simulink model "FSAC2021_V1_Running"  (R2014a)
settings: Solver=FixedStepDiscrete  StartTime=0.0  StopTime=inf  FixedStep=0.0005  RelTol=1e-3
model workspace (MAT data in the model file):
  MCOS : class17 (value not decoded)
  MCOS : class17 (value not decoded)
  MCOS : class17 (value not decoded)
  MCOS : class17 (value not decoded)
  MCOS : class17 (value not decoded)
  MCOS : class17 (value not decoded)
  MCOS : class17 (value not decoded)
  MCOS : class17 (value not decoded)
  MCOS : class17 (value not decoded)
  MCOS : class17 (value not decoded)
  MCOS : class17 (value not decoded)
  MCOS : class17 (value not decoded)
  MCOS : class17 (value not decoded)
  MCOS : class17 (value not decoded)
  MCOS : class17 (value not decoded)
  MCOS : class17 (value not decoded)
  MCOS : class17 (value not decoded)
  MCOS : class17 (value not decoded)
  MCOS : class17 (value not decoded)
  BUZZER_START = 1
  MCOS : class17 (value not decoded)
  MCOS : class17 (value not decoded)
  MCOS : class17 (value not decoded)
  MCOS : class17 (value not decoded)
  MCOS : class17 (value not decoded)
  MCOS : class17 (value not decoded)
  MCOS : class17 (value not decoded)
  MCOS : class17 (value not decoded)
  MCOS : class17 (value not decoded)
  MCOS : class17 (value not decoded)
  MCOS : class17 (value not decoded)
  MCOS : class17 (value not decoded)
  MCOS : class17 (value not decoded)
  MCOS : class17 (value not decoded)
  MCOS : class17 (value not decoded)
  MCOS : class17 (value not decoded)
  MCOS : class17 (value not decoded)
  MCOS : class17 (value not decoded)
  MCOS : class17 (value not decoded)
  MCOS : class17 (value not decoded)
  MCOS : class17 (value not decoded)
  MCOS : class17 (value not decoded)
  MCOS : class17 (value not decoded)
  MCOS : class17 (value not decoded)
  MCOS : class17 (value not decoded)
  MCOS : class17 (value not decoded)
  MCOS : class17 (value not decoded)
  MCOS : class17 (value not decoded)
  MCOS : class17 (value not decoded)
  MCOS : class17 (value not decoded)
  MCOS : class17 (value not decoded)
  MCOS : class17 (value not decoded)
  MCOS : class17 (value not decoded)
  MCOS : class17 (value not decoded)
  MCOS : class17 (value not decoded)
  MCOS : class17 (value not decoded)
  MCOS : class17 (value not decoded)
  MCOS : class17 (value not decoded)
  Brake = 11
  MCOS : class17 (value not decoded)
  MCOS : class17 (value not decoded)
  MCOS : class17 (value not decoded)
  MCOS : class17 (value not decoded)
  MCOS : class17 (value not decoded)
  MCOS : class17 (value not decoded)
  MCOS : class17 (value not decoded)
  MCOS : class17 (value not decoded)
  Sensor_Acc_b = 101.85
  Sensor_Acc_k = -0.0185
  Str_Sen_Orig_Angle = -341
  MCOS : class17 (value not decoded)
  Tire_D = 0.47
  T = 0.05
libraries: simulink x402, ec55xxlib x134
(part 4 of 17)

== system FSAC2021_V1_Running/CAN_SEND/Subsystem1/MOTEC_CONTROL ==
  Fault_Reset_in : Inport
  Position_set_in : Inport  Port=2
  New_Pos_Set_in : Inport  Port=3
  Halt_Ctrl_in : Inport  Port=4
  Abs_or_Rel_Ctrl_in : Inport  Port=5
  Switch_On_Ctrl_in : Inport  Port=6
  Quick_Stop_Ctrl_in : Inport  Port=7
  Enable_Voltage_Ctrl_in : Inport  Port=8
  Enable_Operation_Ctrl_in : Inport  Port=9
  function : TriggerPort  TriggerType=function-call
  Abs_or_Rel_Ctrl : Subsystem
  Conv{1..6} (6 alike) : DataTypeConversion
  Enable_Operation_Ctrl : Subsystem
  Enable_Voltage_Ctrl : Subsystem
  Fault_Reset : Subsystem
  Halt_Ctrl : Subsystem
  MOTEC_CONTROL_mux : Mux  Inputs=6
  New_Pos_Set : Subsystem
  Position_set : Subsystem
  Quick_Stop_Ctrl : Subsystem
  Switch_On_Ctrl : Subsystem
  or1 : simulink/Logic and Bit Operations/Bitwise Operator  logicop=OR  UseBitMask=off  NumInputPorts=7  BitMask=bin2dec('11011001')  BitMaskRealWorld=Stored Integer
  output : Outport
  wires:
  MOTEC_CONTROL_mux/1 -> output/1
  Fault_Reset/1(output1) -> or1/1
  New_Pos_Set/1(output1) -> or1/3
  Abs_or_Rel_Ctrl/1(output1) -> or1/5
  Switch_On_Ctrl/1(output1) -> or1/6
  Quick_Stop_Ctrl/1(output1) -> or1/7
  Enable_Voltage_Ctrl/1(output1) -> or1/2
  Enable_Operation_Ctrl/1(output1) -> or1/4
  or1/1 -> Conv1/1
  Conv1/1 -> MOTEC_CONTROL_mux/1
  Halt_Ctrl/1(output2) -> Conv2/1
  Conv2/1 -> MOTEC_CONTROL_mux/2
  Position_set/1(output3) -> Conv3/1
  Conv3/1 -> MOTEC_CONTROL_mux/3
  Position_set/2(output4) -> Conv4/1
  Conv4/1 -> MOTEC_CONTROL_mux/4
  Position_set/3(output5) -> Conv5/1
  Conv5/1 -> MOTEC_CONTROL_mux/5
  Position_set/4(output6) -> Conv6/1
  Conv6/1 -> MOTEC_CONTROL_mux/6
  Fault_Reset_in/1 -> Fault_Reset/1(Fault_Reset)
  Position_set_in/1 -> Position_set/1(Position_set)
  New_Pos_Set_in/1 -> New_Pos_Set/1(New_Pos_Set)
  Halt_Ctrl_in/1 -> Halt_Ctrl/1(Halt_Ctrl)
  Abs_or_Rel_Ctrl_in/1 -> Abs_or_Rel_Ctrl/1(Abs_or_Rel_Ctrl)
  Switch_On_Ctrl_in/1 -> Switch_On_Ctrl/1(Switch_On_Ctrl)
  Quick_Stop_Ctrl_in/1 -> Quick_Stop_Ctrl/1(Quick_Stop_Ctrl)
  Enable_Voltage_Ctrl_in/1 -> Enable_Voltage_Ctrl/1(Enable_Voltage_Ctrl)
  Enable_Operation_Ctrl_in/1 -> Enable_Operation_Ctrl/1(Enable_Operation_Ctrl)

== system FSAC2021_V1_Running/CAN_SEND/Subsystem1/MOTEC_ENCODER1 ==
  Str_Encoder1_in : Inport
  Str_Encoder2_in : Inport  Port=2
  Str_Encoder3_in : Inport  Port=3
  Str_Encoder4_in : Inport  Port=4
  Str_Encoder5_in : Inport  Port=5
  Str_Encoder6_in : Inport  Port=6
  function : TriggerPort  TriggerType=function-call
  Conv{1..6} (6 alike) : DataTypeConversion
  MOTEC_ENCODER_mux : Mux  Inputs=6
  Str_Encoder1 : Subsystem
  Str_Encoder2 : Subsystem
  Str_Encoder3 : Subsystem
  Str_Encoder4 : Subsystem
  Str_Encoder5 : Subsystem
  Str_Encoder6 : Subsystem
  output : Outport
  wires:
  MOTEC_ENCODER_mux/1 -> output/1
  Str_Encoder1/1(output1) -> Conv1/1
  Conv1/1 -> MOTEC_ENCODER_mux/1
  Str_Encoder2/1(output2) -> Conv2/1
  Conv2/1 -> MOTEC_ENCODER_mux/2
  Conv3/1 -> MOTEC_ENCODER_mux/3
  Str_Encoder4/1(output4) -> Conv4/1
  Conv4/1 -> MOTEC_ENCODER_mux/4
  Str_Encoder5/1(output5) -> Conv5/1
  Conv5/1 -> MOTEC_ENCODER_mux/5
  Str_Encoder6/1(output6) -> Conv6/1
  Conv6/1 -> MOTEC_ENCODER_mux/6
  Str_Encoder4_in/1 -> Str_Encoder4/1(Str_Encoder4)
  Str_Encoder6_in/1 -> Str_Encoder6/1(Str_Encoder6)
  Str_Encoder5_in/1 -> Str_Encoder5/1(Str_Encoder5)
  Str_Encoder3_in/1 -> Str_Encoder3/1(Str_Encoder3)
  Str_Encoder2_in/1 -> Str_Encoder2/1(Str_Encoder2)
  Str_Encoder1_in/1 -> Str_Encoder1/1(Str_Encoder1)
  Str_Encoder3/1(output3) -> Conv3/1

== system FSAC2021_V1_Running/CAN_SEND/Subsystem1/MOTEC_NMT ==
  NMT_nodeorder_in : Inport
  NMT_nodectrl_in : Inport  Port=2
  function : TriggerPort  TriggerType=function-call
  Conv1 : DataTypeConversion
  Conv2 : DataTypeConversion
  MOTEC_NMT_mux : Mux  Inputs=2
  NMT_nodectrl : Subsystem
  NMT_nodeorder : Subsystem
  output : Outport
  wires:
  MOTEC_NMT_mux/1 -> output/1
  NMT_nodeorder/1(output1) -> Conv1/1
  Conv1/1 -> MOTEC_NMT_mux/1
  NMT_nodectrl/1(output2) -> Conv2/1
  Conv2/1 -> MOTEC_NMT_mux/2
  NMT_nodeorder_in/1 -> NMT_nodeorder/1(NMT_nodeorder)
  NMT_nodectrl_in/1 -> NMT_nodectrl/1(NMT_nodectrl)

== system FSAC2021_V1_Running/Controller/200ms_Duty/Light_Subsystem ==
  Light_Status : Inport
  "BLINK " : Subsystem  TreatAsAtomicUnit=on
  Data Type Conversion : DataTypeConversion  OutDataTypeStr=uint8
  If : If  IfExpression=u1 == 0  ElseIfExpressions=u1 == 1
  Merge : Merge  Inputs=3
  OFF : Subsystem  TreatAsAtomicUnit=on
  ON : Subsystem  TreatAsAtomicUnit=on
  Light_Output : Outport
  wires:
  ON/1(Out1) -> Merge/1
  Data Type Conversion/1 -> Light_Output/1
  OFF/1(Out1) -> Merge/2
  Merge/1 -> Data Type Conversion/1
  "BLINK "/1(Out1) -> Merge/3
  Light_Status/1 -> If/1
  If/3 -> "BLINK "/Action
  If/1 -> ON/Action
  If/2 -> OFF/Action

== system FSAC2021_V1_Running/Controller/200ms_Duty/Light_Subsystem1 ==
  Light_Status : Inport
  BLINK : Subsystem  TreatAsAtomicUnit=on
  Data Type Conversion : DataTypeConversion  OutDataTypeStr=uint8
  If : If  IfExpression=u1 == 0  ElseIfExpressions=u1 == 1
  Merge : Merge  Inputs=3
  OFF : Subsystem  TreatAsAtomicUnit=on
  ON : Subsystem  TreatAsAtomicUnit=on
  Light_Output : Outport
  wires:
  If/2 -> OFF/Action
  If/1 -> ON/Action
  If/3 -> BLINK/Action
  Light_Status/1 -> If/1
  BLINK/1(Out1) -> Merge/3
  Merge/1 -> Data Type Conversion/1
  OFF/1(Out1) -> Merge/2
  Data Type Conversion/1 -> Light_Output/1
  ON/1(Out1) -> Merge/1

== system FSAC2021_V1_Running/Controller/200ms_Duty/Light_Subsystem2 ==
  Buzzer_Flag : Inport
  Data Type Conversion : DataTypeConversion  OutDataTypeStr=uint8
  EBS_Horn : Subsystem  TreatAsAtomicUnit=on
  If : If  IfExpression=u1 == 0  ElseIfExpressions=u1 == 1
  Merge : Merge  Inputs=3
  Start_Horn : Subsystem  TreatAsAtomicUnit=on
  off : Subsystem  TreatAsAtomicUnit=on
  Buzzer_Pin : Outport
  Buzzer_Overflag : Outport  Port=2
  wires:
  off/1(Out1) -> Merge/1
  Data Type Conversion/1 -> Buzzer_Pin/1
  Start_Horn/1(Out1) -> Merge/2
  Merge/1 -> Data Type Conversion/1
  EBS_Horn/1(Buzzer_Pin) -> Merge/3
  Buzzer_Flag/1 -> If/1
  If/3 -> EBS_Horn/Action
  If/1 -> off/Action
  If/2 -> Start_Horn/Action
  EBS_Horn/2(Buzzer_Overflag) -> Buzzer_Overflag/1

== system FSAC2021_V1_Running/Controller/50ms_Duty/48Battry_Judge ==
  note: 1.OPEN
      | 0.CLOSE
  Str_Sys_Error : Inport
  Brk_Sys_Error : Inport  Port=2
  AS_48V_Relay : Inport  Port=3
  Logical Operator : Logic  AllPortsSameDT=off  OutDataTypeStr=boolean
  Logical Operator2 : Logic  Operator=OR  AllPortsSameDT=off  OutDataTypeStr=boolean
  Logical Operator3 : Logic  Operator=NOT  Inputs=1  AllPortsSameDT=off  OutDataTypeStr=boolean
  Relay_48V_Pin : Outport
  wires:
  AS_48V_Relay/1 -> Logical Operator/2
  Logical Operator/1 -> Relay_48V_Pin/1
  Str_Sys_Error/1 -> Logical Operator2/1
  Brk_Sys_Error/1 -> Logical Operator2/2
  Logical Operator2/1 -> Logical Operator3/1
  Logical Operator3/1 -> Logical Operator/1

== system FSAC2021_V1_Running/Controller/50ms_Duty/EBS_Judge ==
  note: 0 :disable
  note: 1 :armed
  note: 2 :enable
      |
      | 3: No mean
  EBS_GAS_Prs_1_Val : Inport
  EBS_GAS_Prs_2_Val : Inport  Port=2
  Brk_Liquid_Prs_Val : Inport  Port=3
  Constant : Constant  Value=0.4  OutDataTypeStr=single
  Constant1 : Constant  Value=0.4  OutDataTypeStr=single
  Constant2 : Constant  Value=2.8  OutDataTypeStr=single
  Relational Operator : RelationalOperator  Operator=<=  OutDataTypeStr=boolean
  Relational Operator1 : RelationalOperator  Operator=<=  OutDataTypeStr=boolean
  Relational Operator2 : RelationalOperator  Operator=<=  OutDataTypeStr=boolean
  Truth Table : Truth Table  TreatAsAtomicUnit=on
  EBS_Status : Outport
  wires:
  EBS_GAS_Prs_1_Val/1 -> Relational Operator/1
  Constant/1 -> Relational Operator/2
  Constant1/1 -> Relational Operator1/2
  EBS_GAS_Prs_2_Val/1 -> Relational Operator1/1
  Relational Operator/1 -> Truth Table/1(Gas_1_Flag)  "0:No gas;1 Has gas"
  Relational Operator1/1 -> Truth Table/2(Gas_2_Flag)  "0:No gas;1 Has gas"
  Brk_Liquid_Prs_Val/1 -> Relational Operator2/1
  Constant2/1 -> Relational Operator2/2
  Relational Operator2/1 -> Truth Table/3(Liquid_Flag)  "0:No Brk;1 Has Brk"
  Truth Table/1(EBS_Status) -> EBS_Status/1

== system FSAC2021_V1_Running/Controller/50ms_Duty/HV_Judge  ==
  HV_LIGHT : Inport
  HVMS : Inport  Port=2
  ON_OUT : Inport  Port=3
  ON_IN : Inport  Port=4
  Compare_Volt_mv : Inport  Port=5
  Compare To Constant : simulink/Logic and Bit Operations/Compare To Constant  relop=>=  const=2  OutDataTypeStr=boolean
  Data Type Conversion : DataTypeConversion  OutDataTypeStr=uint8
  Logical Operator : Logic  Inputs=3  AllPortsSameDT=off  OutDataTypeStr=boolean
  Logical Operator1 : Logic  Operator=OR  AllPortsSameDT=off  OutDataTypeStr=boolean
  Logical Operator4 : Logic  AllPortsSameDT=off  OutDataTypeStr=boolean
  MeaModule : ec55xxlib/RapidECU_U2/11Calibration/MeaModule  signal=Compare_Voltage
  TS_Flag : Outport
  wires:
  HVMS/1 -> Logical Operator/2
  ON_OUT/1 -> Logical Operator1/1
  Logical Operator1/1 -> Logical Operator/3
  Logical Operator/1 -> Logical Operator4/2
  Logical Operator4/1 -> Data Type Conversion/1
  Data Type Conversion/1 -> TS_Flag/1
  ON_IN/1 -> Logical Operator1/2
  HV_LIGHT/1 -> Logical Operator/1
  Compare To Constant/1 -> MeaModule/1
  MeaModule/1 -> Logical Operator4/1
  Compare_Volt_mv/1 -> Compare To Constant/1

== system FSAC2021_V1_Running/Controller/50ms_Duty/Lights_Select ==
  Visual_Lights_Vetor : Inport
  Visual_Flag : Inport  Port=2
  IMD_Error : Inport  Port=3
  EBS_Error : Inport  Port=4
  BMS_Error : Inport  Port=5
  Demux : Demux  Outputs=3
  Mux : Mux  Inputs=3
  Switch : Switch  Criteria=u2 > Threshold
  IMD_Light_Sts : Outport
  EBS_Light_Sts : Outport  Port=2
  BMS_Light_Sts : Outport  Port=3
  wires:
  BMS_Error/1 -> Mux/3
  Visual_Flag/1 -> Switch/2
  Visual_Lights_Vetor/1 -> Switch/1
  EBS_Error/1 -> Mux/2
  Mux/1 -> Switch/3
  IMD_Error/1 -> Mux/1
  Switch/1 -> Demux/1
  Demux/1 -> IMD_Light_Sts/1
  Demux/2 -> EBS_Light_Sts/1
  Demux/3 -> BMS_Light_Sts/1

== system FSAC2021_V1_Running/Controller/50ms_Duty/R2D_Judge ==
  AS_R2D : Inport
  Acc_Sensor_Error : Inport  Port=2
  Logical Operator : Logic  AllPortsSameDT=off  OutDataTypeStr=boolean
  Logical Operator1 : Logic  Operator=NOT  Inputs=1  AllPortsSameDT=off  OutDataTypeStr=boolean
  R2D_Pin : Outport
  wires:
  Logical Operator/1 -> R2D_Pin/1
  AS_R2D/1 -> Logical Operator/1
  Acc_Sensor_Error/1 -> Logical Operator1/1
  Logical Operator1/1 -> Logical Operator/2

== system FSAC2021_V1_Running/Controller/50ms_Duty/Safety_Relay_Judge ==
  note: 0:Disable
      | 1:Armed
      | 2:Enable
  Finish_State_Safety_Relay : Inport
  Str_Sys_Error : Inport  Port=2
  Brk_Sys_Error : Inport  Port=3
  Sensor_Error : Inport  Port=4
  Node_Lost : Inport  Port=5
  EBS_Failure : Inport  Port=6
  Logical Operator : Logic  Operator=OR  Inputs=6  AllPortsSameDT=off  OutDataTypeStr=boolean
  Safety_Cir_Relay_Pin : Outport
  wires:
  Logical Operator/1 -> Safety_Cir_Relay_Pin/1
  Finish_State_Safety_Relay/1 -> Logical Operator/1
  EBS_Failure/1 -> Logical Operator/6
  Node_Lost/1 -> Logical Operator/5
  Sensor_Error/1 -> Logical Operator/4
  Brk_Sys_Error/1 -> Logical Operator/3
  Str_Sys_Error/1 -> Logical Operator/2

== system FSAC2021_V1_Running/Controller/50ms_Duty/Subsystem ==
  note: TASK:
      | 1、SKIDPAD
      | 2、ACCELERATION
      | 3、TRACKDRIVE
      | 4、BRAKTEST
      | 5、INSPECTION
      | 6、MANUAL_MODE
  Manual_Acc_Cmd : Inport
  AMI_Duty : Inport  Port=2
  IPC_Acc_Cmd : Inport  Port=3
  EBS_Failure : Inport  Port=4
  IPC_Brk_Cmd : Inport  Port=5
  IPC_Str_Cmd : Inport  Port=6
  origin_flag : Inport  Port=7
  ASSI_State : Inport  Port=8
  Allow_Ctr_Flag : Inport  Port=9
  Chart : Stateflow chart  TreatAsAtomicUnit=on
  Compare To Constant : simulink/Logic and Bit Operations/Compare To Constant  relop===  const=1  OutDataTypeStr=boolean
  Compare To Constant1 : simulink/Logic and Bit Operations/Compare To Constant  relop===  const=2  OutDataTypeStr=boolean
  Compare To Constant2 : simulink/Logic and Bit Operations/Compare To Constant  relop===  const=3  OutDataTypeStr=boolean
  Compare To Constant3 : simulink/Logic and Bit Operations/Compare To Constant  relop===  const=1  OutDataTypeStr=boolean
  Compare To Constant4 : simulink/Logic and Bit Operations/Compare To Constant  relop===  const=1  OutDataTypeStr=boolean
  Compare To Constant5 : simulink/Logic and Bit Operations/Compare To Constant  relop=>=  const=3  OutDataTypeStr=boolean
  Constant : Constant
  Data Type Conversion10 : DataTypeConversion  OutDataTypeStr=single
  Data Type Conversion9 : DataTypeConversion  OutDataTypeStr=uint8
  Logical Operator : Logic  Inputs=4  AllPortsSameDT=off  OutDataTypeStr=boolean
  Logical Operator1 : Logic  AllPortsSameDT=off  OutDataTypeStr=boolean
  MeaModule : ec55xxlib/RapidECU_U2/11Calibration/MeaModule  signal=MODE
  MeaModule1 : ec55xxlib/RapidECU_U2/11Calibration/MeaModule  signal=enable
  MeaModule3 : ec55xxlib/RapidECU_U2/11Calibration/MeaModule  signal=ipc_strr
  Merge : Merge  Inputs=3
  Merge1 : Merge
  Subsystem : Subsystem
  Subsystem1 : Subsystem
  Subsystem2 : Subsystem
  Str_Ctr : Outport
  Brk_Ctr : Outport  Port=2
  Mission_Flag : Outport  Port=3
  Acc_Ctr : Outport  Port=4
  wires:
  Data Type Conversion9/1 -> Brk_Ctr/1
  AMI_Duty/1 -> Chart/1(AMI_Duty)
  Chart/1(MODE) -> MeaModule/1
  MeaModule/1 -> Compare To Constant/1, Compare To Constant1/1, Compare To Constant2/1
  Manual_Acc_Cmd/1 -> Subsystem/1(acc)
  Compare To Constant/1 -> Subsystem/Enable
  EBS_Failure/1 -> Subsystem1/2(EBS_Failure)
  IPC_Brk_Cmd/1 -> Subsystem1/3(IPC_Brk_Cmd)
  IPC_Str_Cmd/1 -> Subsystem1/4(IPC_Str_Cmd)
  IPC_Acc_Cmd/1 -> Subsystem1/1(IPC_Acc_Cmd)
  Subsystem1/1(Brk_Cmd) -> Data Type Conversion9/1
  Compare To Constant2/1 -> Logical Operator/1
  Compare To Constant4/1 -> Logical Operator/2
  origin_flag/1 -> Compare To Constant4/1
  Merge1/1 -> Str_Ctr/1
  Logical Operator/1 -> MeaModule1/1
  Subsystem2/1(ACC) -> [Task_Acc]
  Compare To Constant1/1 -> Logical Operator1/1
  Logical Operator1/1 -> Subsystem1/Enable
  Compare To Constant3/1 -> Logical Operator/3
  Constant/1 -> Compare To Constant3/1, Logical Operator1/2
  Subsystem1/3(Acc_Cmd) -> [IPC_Acc_Cmd]
  Subsystem/1(Acc_Cmd) -> [Manual_Acc]
  Data Type Conversion10/1 -> Acc_Ctr/1
  Merge/1 -> Data Type Conversion10/1
  [IPC_Acc_Cmd] -> Merge/1
  [Manual_Acc] -> Merge/2
  [Task_Acc] -> Merge/3
  Subsystem1/2(Str_Cmd) -> [IPC_Str_Cmd]
  Subsystem2/2(SteerCmd) -> [Task_Steer_Cmd]
  [IPC_Str_Cmd] -> MeaModule3/1
  MeaModule1/1 -> Subsystem2/Enable
  MeaModule3/1 -> Merge1/1
  [Task_Steer_Cmd] -> Merge1/2
  Subsystem2/3(Mission_Flag) -> Mission_Flag/1
  Compare To Constant5/1 -> Logical Operator/4
  ASSI_State/1 -> Compare To Constant5/1

== system FSAC2021_V1_Running/Controller/50ms_Duty/Visuality Check ==
  function : TriggerPort  TriggerType=function-call
  Chart : Stateflow chart  TreatAsAtomicUnit=on
  Visual_Lights_Vector : Outport
  Visual_Flag : Outport  Port=2
  wires:
  Chart/1(Visual_Lights) -> Visual_Lights_Vector/1
  Chart/2(Visual_Flag) -> Visual_Flag/1

== system FSAC2021_V1_Running/Controller/BCU_Controller/Brk_Move ==
  Brk_Ctrl_State : Inport
  Brk_Cmd : Inport  Port=2
  Constant : Constant  Value=BRK_ENGAGED
  Constant1 : Constant  Value=BRK_TOZERO
  Constant2 : Constant  Value=BRK_MOVE
  Enabled Subsystem : Subsystem  TreatAsAtomicUnit=on
  Enabled Subsystem1 : Subsystem  TreatAsAtomicUnit=on
  Enabled Subsystem2 : Subsystem  TreatAsAtomicUnit=on
  Equal : RelationalOperator  Operator===  OutDataTypeStr=boolean
  Equal1 : RelationalOperator  Operator===  OutDataTypeStr=boolean
  Equal2 : RelationalOperator  Operator===  OutDataTypeStr=boolean
  Multiport Switch : MultiPortSwitch  DiagnosticForDefault=None
  Brk_Mtr_GoalPos : Outport
  tag scope: Engaged_Angle=global
  wires:
  [Engaged_Angle] -> Enabled Subsystem1/1(Engaged_Angle)
  Enabled Subsystem/2(Engaged_Angle) -> [Engaged_Angle]
  Brk_Cmd/1 -> Enabled Subsystem2/1(Brk_Prop)
  Enabled Subsystem2/1(Move_Pulses) -> Multiport Switch/4
  Enabled Subsystem1/1(ToZero_Pulses) -> Multiport Switch/3
  Enabled Subsystem/1(Engaged_Pulses) -> Multiport Switch/2
  Equal2/1 -> Enabled Subsystem2/Enable
  Equal1/1 -> Enabled Subsystem1/Enable
  Equal/1 -> Enabled Subsystem/Enable
  Constant2/1 -> Equal2/2
  Constant1/1 -> Equal1/2
  Constant/1 -> Equal/2
  Brk_Ctrl_State/1 -> Multiport Switch/1, Equal/1, Equal1/1, Equal2/1
  Multiport Switch/1 -> Brk_Mtr_GoalPos/1

== system FSAC2021_V1_Running/Controller/SteerCtr/Subsystem3 ==
  In1 : Inport
  Constant : Constant  Value=Str_Sen_Orig_Angle  OutDataTypeStr=int16
  Real_steer_angle : Sum  Inputs=+-  OutDataTypeStr=single
  Out1 : Outport
  wires:
  Real_steer_angle/1 -> Out1/1
  In1/1 -> Real_steer_angle/1
  Constant/1 -> Real_steer_angle/2

== system FSAC2021_V1_Running/DIAG/DIAG/Analog_Sensor_Diag ==
  Acc_Lft_Disp_mv : Inport
  Acc_Right_Disp_mv : Inport  Port=2
  Brk_Liquid_Prs_mv : Inport  Port=3
  EBS_GAS_Prs_1_mv : Inport  Port=4
  EBS_GAS_Prs_2_mv : Inport  Port=5
  Chart2 : Stateflow chart  TreatAsAtomicUnit=on
      settings: RTWSystemCode=Reusable function
  Chart3 : Stateflow chart  TreatAsAtomicUnit=on
      settings: RTWSystemCode=Reusable function
  Chart4 : Stateflow chart  TreatAsAtomicUnit=on
      settings: RTWSystemCode=Reusable function
  Chart5 : Stateflow chart  TreatAsAtomicUnit=on
      settings: RTWSystemCode=Reusable function
  Chart6 : Stateflow chart  TreatAsAtomicUnit=on
      settings: RTWSystemCode=Reusable function
  Compare To Constant{,1..4} (5 alike) : simulink/Logic and Bit Operations/Compare To Constant  relop=<=  const=Min  OutDataTypeStr=boolean
  Data Type Conversion{1..5} (5 alike) : DataTypeConversion  OutDataTypeStr=uint8
  Logical Operator8 : Logic  Operator=OR  Inputs=5  AllPortsSameDT=off  OutDataTypeStr=boolean
  MeaModule : ec55xxlib/RapidECU_U2/11Calibration/MeaModule  signal=sensor_erroe
  Acc_Lft_Error : Outport
  Acc_Right_Disp_Error : Outport  Port=2
  Brk_Liquid_Prs_Error : Outport  Port=3
  Sensor_Error : Outport  Port=4
  EBS_GAP_pRS_1_Error : Outport  Port=5
  EBS_GAP_pRS_2_Error : Outport  Port=6
  wires:
  EBS_GAS_Prs_1_mv/1 -> Compare To Constant3/1
  Acc_Lft_Disp_mv/1 -> Compare To Constant/1
  Acc_Right_Disp_mv/1 -> Compare To Constant1/1
  EBS_GAS_Prs_2_mv/1 -> Compare To Constant4/1
  Logical Operator8/1 -> MeaModule/1
  Chart2/1(Debounce) -> Acc_Lft_Error/1, Logical Operator8/1
  Chart3/1(Debounce) -> Acc_Right_Disp_Error/1, Logical Operator8/2
  Chart4/1(Debounce) -> Brk_Liquid_Prs_Error/1, Logical Operator8/3
  Chart5/1(Debounce) -> Logical Operator8/4, EBS_GAP_pRS_1_Error/1
  Chart6/1(Debounce) -> Logical Operator8/5, EBS_GAP_pRS_2_Error/1
  Data Type Conversion1/1 -> Chart2/1(Non_Debounce)
  Data Type Conversion2/1 -> Chart3/1(Non_Debounce)
  Data Type Conversion3/1 -> Chart4/1(Non_Debounce)
  Data Type Conversion4/1 -> Chart5/1(Non_Debounce)
  Data Type Conversion5/1 -> Chart6/1(Non_Debounce)
  Brk_Liquid_Prs_mv/1 -> Compare To Constant2/1
  Compare To Constant1/1 -> Data Type Conversion2/1
  Compare To Constant/1 -> Data Type Conversion1/1
  Compare To Constant2/1 -> Data Type Conversion3/1
  Compare To Constant3/1 -> Data Type Conversion4/1
  Compare To Constant4/1 -> Data Type Conversion5/1
  MeaModule/1 -> Sensor_Error/1

== system FSAC2021_V1_Running/DIAG/DIAG/BMS_Diag ==
  ALM_BATT_OC_Out1 : Inport
  ALM_AUX_FAIL_Out1 : Inport  Port=2
  ALM_BATT_UV_Out1 : Inport  Port=3
  ALM_BATT_OV_Out1 : Inport  Port=4
  ALM_BATT_DT_Out1 : Inport  Port=5
  ALM_BATT_DV_Out1 : Inport  Port=6
  ALM_CELL_TBK_Out1 : Inport  Port=7
  ALM_CELL_IBK_Out1 : Inport  Port=8
  ALM_CELL_UT_Out1 : Inport  Port=9
  ALM_CELL_OT_Out1 : Inport  Port=10
  ALM_CELL_UV_Out1 : Inport  Port=11
  ALM_CELL_OV_Out1 : Inport  Port=12
  ALM_BATT_UC_Out1 : Inport  Port=13
  ALM_PRECHRG_FAIL_Out1 : Inport  Port=14
  ALM_LEAK_OC_Out1 : Inport  Port=15
  ALM_HVREL_FAIL_Out1 : Inport  Port=16
  ALM_HALL_BREAK_Out1 : Inport  Port=17
  ALM_BSU_OFFLINE_Out1 : Inport  Port=18
  ALM_BSU_FAULT_Out1 : Inport  Port=19
  ALM_BMU_FAIL_Out1 : Inport  Port=20
  Data Type Conversion{,1..16,19,22..23} (20 alike) : DataTypeConversion  OutDataTypeStr=boolean  SaturateOnIntegerOverflow=on  RndMeth=Zero
  Data Type Conversion17 : DataTypeConversion  OutDataTypeStr=uint8
  Logical Operator : Logic  Operator=OR  Inputs=20  AllPortsSameDT=off  OutDataTypeStr=boolean
  "BMS_Error " : Outport
  wires:
  ALM_BATT_OC_Out1/1 -> Data Type Conversion/1
  ALM_BATT_DT_Out1/1 -> Data Type Conversion1/1
  ALM_AUX_FAIL_Out1/1 -> Data Type Conversion2/1
  ALM_BATT_UV_Out1/1 -> Data Type Conversion3/1
  ALM_BATT_OV_Out1/1 -> Data Type Conversion4/1
  ALM_CELL_TBK_Out1/1 -> Data Type Conversion5/1
  ALM_CELL_UV_Out1/1 -> Data Type Conversion6/1
  ALM_CELL_UT_Out1/1 -> Data Type Conversion7/1
  ALM_CELL_IBK_Out1/1 -> Data Type Conversion8/1
  ALM_BATT_DV_Out1/1 -> Data Type Conversion9/1
  ALM_CELL_OT_Out1/1 -> Data Type Conversion10/1
  ALM_BATT_UC_Out1/1 -> Data Type Conversion11/1
  ALM_CELL_OV_Out1/1 -> Data Type Conversion12/1
  ALM_PRECHRG_FAIL_Out1/1 -> Data Type Conversion13/1
  ALM_LEAK_OC_Out1/1 -> Data Type Conversion14/1
  ALM_HVREL_FAIL_Out1/1 -> Data Type Conversion15/1
  ALM_HALL_BREAK_Out1/1 -> Data Type Conversion16/1
  ALM_BSU_OFFLINE_Out1/1 -> Data Type Conversion19/1
  ALM_BMU_FAIL_Out1/1 -> Data Type Conversion22/1
  ALM_BSU_FAULT_Out1/1 -> Data Type Conversion23/1
  Data Type Conversion3/1 -> Logical Operator/11
  Data Type Conversion4/1 -> Logical Operator/12
  Data Type Conversion2/1 -> Logical Operator/10
  Data Type Conversion1/1 -> Logical Operator/13
  Data Type Conversion/1 -> Logical Operator/9
  Data Type Conversion11/1 -> Logical Operator/8
  Data Type Conversion9/1 -> Logical Operator/14
  Data Type Conversion5/1 -> Logical Operator/15
  Data Type Conversion22/1 -> Logical Operator/7
  Data Type Conversion23/1 -> Logical Operator/6
  Data Type Conversion8/1 -> Logical Operator/16
  Data Type Conversion16/1 -> Logical Operator/4
  Data Type Conversion7/1 -> Logical Operator/17
  Data Type Conversion19/1 -> Logical Operator/5
  Data Type Conversion10/1 -> Logical Operator/18
  Data Type Conversion15/1 -> Logical Operator/3
  Data Type Conversion6/1 -> Logical Operator/19
  Data Type Conversion14/1 -> Logical Operator/2
  Data Type Conversion13/1 -> Logical Operator/1
  Data Type Conversion12/1 -> Logical Operator/20
  Logical Operator/1 -> Data Type Conversion17/1
  Data Type Conversion17/1 -> "BMS_Error "/1

== system FSAC2021_V1_Running/DIAG/DIAG/Brake_System_Diag ==
  Brake_reg_rw_fault_flag_Out : Inport
  Brake_overheat_prtct_sts_Out : Inport  Port=2
  Brake_overcurrt_prtct_sts_Out : Inport  Port=3
  Brake_lowvolt_prtct_sts_Out : Inport  Port=4
  Brake_hd_fault_sts_Out : Inport  Port=5
  Brake_encoder_fault_sts_Out : Inport  Port=6
  Brake_cmd_fault_flag_Out : Inport  Port=7
  Logical Operator : Logic  Operator=OR  Inputs=7  AllPortsSameDT=off  OutDataTypeStr=boolean
  Brk_Sys_Error : Outport
  wires:
  Brake_cmd_fault_flag_Out/1 -> Logical Operator/7
  Brake_hd_fault_sts_Out/1 -> Logical Operator/5
  Brake_encoder_fault_sts_Out/1 -> Logical Operator/6
  Brake_overheat_prtct_sts_Out/1 -> Logical Operator/2
  Brake_reg_rw_fault_flag_Out/1 -> Logical Operator/1
  Brake_lowvolt_prtct_sts_Out/1 -> Logical Operator/4
  Brake_overcurrt_prtct_sts_Out/1 -> Logical Operator/3
  Logical Operator/1 -> Brk_Sys_Error/1

== system FSAC2021_V1_Running/DIAG/DIAG/CAN_NODE_LOSTCOM ==
  Brake_Node : Inport
  StrSr_Node : Inport  Port=2
  48V_Relay : Inport  Port=3
  RES_Node : Inport  Port=4
  BMS_Node : Inport  Port=5
  Motor_Node : Inport  Port=6
  Motec_Node : Inport  Port=7
  AMI_Node : Inport  Port=8
  ASSI_State : Inport  Port=9
  B_M_S_Check : Subsystem
  Compare To Constant : simulink/Logic and Bit Operations/Compare To Constant  relop=>=  const=3.0  OutDataTypeStr=boolean
  Compare To Constant1 : simulink/Logic and Bit Operations/Compare To Constant  relop=<=  const=5  OutDataTypeStr=boolean
  Constant : Constant
  Constant1 : Constant
  Constant2 : Constant
  Logical Operator : Logic  Inputs=3  AllPortsSameDT=off  OutDataTypeStr=boolean
  Logical Operator1 : Logic  AllPortsSameDT=off  OutDataTypeStr=boolean
  Logical Operator3 : Logic  Operator=NOT  AllPortsSameDT=off  OutDataTypeStr=boolean
  MeaModule : ec55xxlib/RapidECU_U2/11Calibration/MeaModule  signal=Node_Lost
  Subsystem : Subsystem
  Subsystem1 : Subsystem
  Switch : Switch  Criteria=u2 > Threshold
  Switch1 : Switch  Criteria=u2 > Threshold
  Node_Lost_Flag : Outport
  wires:
  Brake_Node/1 -> B_M_S_Check/1(Brake_Node)
  48V_Relay/1 -> Switch/2, B_M_S_Check/Enable
  B_M_S_Check/1(Node_Lost_Flag) -> Switch/1
  Logical Operator3/1 -> MeaModule/1
  Motec_Node/1 -> B_M_S_Check/2(Motec_Node)
  Constant/1 -> B_M_S_Check/3(RES_Node)
  MeaModule/1 -> Node_Lost_Flag/1
  Motor_Node/1 -> Subsystem/1(Motor_Node)
  Subsystem/1(Node_Lost_Flag) -> Switch1/1
  Constant1/1 -> Switch1/3
  Constant2/1 -> Switch/3
  ASSI_State/1 -> Compare To Constant/1, Compare To Constant1/1
  Switch/1 -> Logical Operator/1
  Logical Operator1/1 -> Subsystem/Enable, Switch1/2
  Compare To Constant/1 -> Logical Operator1/1
  Compare To Constant1/1 -> Logical Operator1/2
  Logical Operator/1 -> Logical Operator3/1
  StrSr_Node/1 -> Subsystem1/1(StrSr_Node)
  BMS_Node/1 -> Subsystem1/2(BMS_Node)
  AMI_Node/1 -> Subsystem1/3(AMI_Node)
  Switch1/1 -> Logical Operator/3
  Subsystem1/1(Out1) -> Logical Operator/2

== system FSAC2021_V1_Running/DIAG/DIAG/EBS_Diag ==
  ASSI_State : Inport
  EBS_GAS_Prs_1_Val : Inport  Port=2  OutDataTypeStr=uint16
  EBS_GAS_Prs_2_Val : Inport  Port=3  OutDataTypeStr=uint16
  Truth Table : Truth Table  TreatAsAtomicUnit=on
  EBS_Failuer_Flag : Outport
  wires:
  ASSI_State/1 -> Truth Table/1(ASSI_State)
  Truth Table/1(EBS_Failure_Flag) -> EBS_Failuer_Flag/1
  EBS_GAS_Prs_1_Val/1 -> Truth Table/2(EBS_GAS_Prs_1_Val)
  EBS_GAS_Prs_2_Val/1 -> Truth Table/3(EBS_GAS_Prs_2_Val)

== system FSAC2021_V1_Running/DIAG/DIAG/Res_Diag ==
  RES_SINGNAL : Inport
  ASMS : Inport  Port=2
  MeaModule : ec55xxlib/RapidECU_U2/11Calibration/MeaModule  signal=ASMS_VALUE
  MeaModule1 : ec55xxlib/RapidECU_U2/11Calibration/MeaModule  signal=res_go
  MeaModule2 : ec55xxlib/RapidECU_U2/11Calibration/MeaModule  signal=res_ebs1
  Subsystem : Subsystem
  Res_Go : Outport
  RES_EBS : Outport  Port=2
  wires:
  Subsystem/1(RES_GO) -> MeaModule1/1
  ASMS/1 -> MeaModule/1
  MeaModule/1 -> Subsystem/Enable
  RES_SINGNAL/1 -> Subsystem/1(RES_SINGNAL)
  Subsystem/2(RES_EBS) -> MeaModule2/1
  MeaModule1/1 -> Res_Go/1
  MeaModule2/1 -> RES_EBS/1

== system FSAC2021_V1_Running/DIAG/DIAG/Steer_System_Diag ==
  Str_UnderVolt_Warning_Out : Inport
  Str_System_Error_Out : Inport  Port=2
  Str_Limit_Pos_Alarm_Out : Inport  Port=3
  Str_I2t_Warning_Out : Inport  Port=4
  Str_I2t_Alarm_Out : Inport  Port=5
  Str_Flash_Error_Out : Inport  Port=6
  Str_Encoder_Error_Out : Inport  Port=7
  Str_Curr_Error_Fault_Out : Inport  Port=8
  Str_Spd_Over_Alam_Out : Inport  Port=9
  Str_PwrMod_TempHigh_Warning_Out : Inport  Port=10
  Str_PwrMod_TempHigh_Alarm_Out : Inport  Port=11
  Str_Para_Error_Out : Inport  Port=12
  Str_Overvolt_Warning_Out : Inport  Port=13
  Str_Over_TopCurr_Out : Inport  Port=14
  Str_Over_SpdError_Out : Inport  Port=15
  Str_Over_PosError_Out : Inport  Port=16
  Logical Operator : Logic  Operator=OR  Inputs=16  AllPortsSameDT=off  OutDataTypeStr=boolean
  Str_Sys_Error : Outport
  wires:
  Str_UnderVolt_Warning_Out/1 -> Logical Operator/1
  Str_System_Error_Out/1 -> Logical Operator/2
  Str_Spd_Over_Alam_Out/1 -> Logical Operator/3
  Str_PwrMod_TempHigh_Warning_Out/1 -> Logical Operator/4
  Str_Limit_Pos_Alarm_Out/1 -> Logical Operator/11
  Str_I2t_Warning_Out/1 -> Logical Operator/12
  Str_PwrMod_TempHigh_Alarm_Out/1 -> Logical Operator/5
  Str_Over_SpdError_Out/1 -> Logical Operator/9
  Str_Overvolt_Warning_Out/1 -> Logical Operator/7
  Str_Para_Error_Out/1 -> Logical Operator/6
  Str_Over_PosError_Out/1 -> Logical Operator/10
  Str_I2t_Alarm_Out/1 -> Logical Operator/13
  Str_Over_TopCurr_Out/1 -> Logical Operator/8
  Str_Flash_Error_Out/1 -> Logical Operator/14
  Str_Encoder_Error_Out/1 -> Logical Operator/15
  Str_Curr_Error_Fault_Out/1 -> Logical Operator/16
  Logical Operator/1 -> Str_Sys_Error/1

== system FSAC2021_V1_Running/DIAG/DIAG/TS_Diag ==
  ASSI_State : Inport
  Compare_Volt_mv : Inport  Port=2
  Compare To Constant : simulink/Logic and Bit Operations/Compare To Constant  relop===  const=2  OutDataTypeStr=boolean
  Compare To Constant1 : simulink/Logic and Bit Operations/Compare To Constant  relop===  const=3  OutDataTypeStr=boolean
  Compare To Constant2 : simulink/Logic and Bit Operations/Compare To Constant  relop===  const=6  OutDataTypeStr=boolean
  Merge : Merge  Inputs=3
  Subsystem : Subsystem  TreatAsAtomicUnit=on
  Subsystem1 : Subsystem  TreatAsAtomicUnit=on
  Subsystem2 : Subsystem  TreatAsAtomicUnit=on
  TS_Error : Outport
  wires:
  ASSI_State/1 -> Compare To Constant/1, Compare To Constant2/1, Compare To Constant1/1
  Compare To Constant2/1 -> Subsystem2/Enable
  Subsystem/1(TS_Error) -> Merge/1
  Compare To Constant/1 -> Subsystem/Enable
  Compare To Constant1/1 -> Subsystem1/Enable
  Merge/1 -> TS_Error/1
  Compare_Volt_mv/1 -> Subsystem2/1(Compare_Volt_mv), Subsystem1/1(Compare_Volt_mv), Subsystem/1(Compare_Volt_mv)
  Subsystem1/1(TS_Error) -> Merge/2
  Subsystem2/1(TS_Error) -> Merge/3

== system FSAC2021_V1_Running/DIAG/DIAG/TS_Diag1 ==
  "IMD_BMS " : Inport
  "IMD_BENDER " : Inport  Port=2
  Data Type Conversion : DataTypeConversion  OutDataTypeStr=uint8
  Logical Operator : Logic  AllPortsSameDT=off  OutDataTypeStr=boolean
  IMD_Error : Outport
  wires:
  "IMD_BMS "/1 -> Logical Operator/1
  "IMD_BENDER "/1 -> Logical Operator/2
  Logical Operator/1 -> Data Type Conversion/1
  Data Type Conversion/1 -> IMD_Error/1

== system FSAC2021_V1_Running/Input_Process/KL_Sig_Process/Analog_Signal_Process ==
  note: 0-1500r
  note: 0-Cabli(MPa)
  note: 0-Cabli(MPa)
  note: 0-Cabli(MPa)
  note: 0-100%
  note: 0-100%
  note: 制动压力传感器0-5V对应0-5MPa
      | 制动液压：y=0.001x
  note: EBS压力传感器：0-3.3v 对应 0-1.6Mpa
      |
      | y=0.000303x
  note: 左边传感器：O=0.045i-90
  note: 右边传感器：O=-0.042i+100.8
  Acc_Lft_Disp_mv : Inport
  Acc_Right_Disp_mv : Inport  Port=2
  Brk_Liquid_Prs_mv : Inport  Port=3
  EBS_GAS_Prs_1_mv : Inport  Port=4
  EBS_GAS_Prs_2_mv : Inport  Port=5
  Acc_Lft_Offset : Constant  Value=Acc_Lft_Offset
  Acc_Right_Offset : Constant  Value=408.33
  Add{,1,3..5} (5 alike) : Sum
  Brk_Liquid_Prs_Factor : Constant  Value=Brk_Liquid_Prs_Factor
  Brk_Liquid_Prs_Offset : Constant  Value=Brk_Liquid_Prs_Offset
  Constant : Constant  Value=Acc_Left_Factor
  Constant1 : Constant  Value=-0.08333
  Divide{,1,3..5} (5 alike) : Product  Inputs=**
  EBS_GAS_Prs_1_Factor : Constant  Value=EBS_Prs_Factor
  EBS_GAS_Prs_2_Factor : Constant  Value=EBS_Prs_Factor
  EBS_Prs_Offset : Constant  Value=EBS_Prs_Offset
  EBS_Prs_Offset1 : Constant  Value=EBS_Prs_Offset
  Gain : Gain  Gain=15
  Saturation : Saturate  UpperLimit=100  LowerLimit=0
  Saturation1 : Saturate  UpperLimit=100  LowerLimit=0
  Saturation2 : Saturate  UpperLimit=1500  LowerLimit=0
  Acc_Lft_Disp_Val : Outport
  Acc_Right_Disp_Val : Outport  Port=2
  Brk_Liquid_Prs_Val : Outport  Port=3
  EBS_GAS_Prs_1_Val : Outport  Port=4
  EBS_GAS_Prs_2_Val : Outport  Port=5
  wires:
  Saturation/1 -> Acc_Lft_Disp_Val/1
  Saturation1/1 -> Gain/1
  Add3/1 -> Brk_Liquid_Prs_Val/1
  Add4/1 -> EBS_GAS_Prs_1_Val/1
  Add5/1 -> EBS_GAS_Prs_2_Val/1
  Acc_Right_Offset/1 -> Add1/2
  Constant1/1 -> Divide1/2
  Acc_Lft_Offset/1 -> Add/2
  Divide5/1 -> Add5/1
  EBS_Prs_Offset/1 -> Add5/2
  EBS_GAS_Prs_2_Factor/1 -> Divide5/2
  EBS_GAS_Prs_2_mv/1 -> Divide5/1
  Divide3/1 -> Add3/1
  Divide4/1 -> Add4/1
  EBS_Prs_Offset1/1 -> Add4/2
  EBS_GAS_Prs_1_Factor/1 -> Divide4/2
  EBS_GAS_Prs_1_mv/1 -> Divide4/1
  Brk_Liquid_Prs_Offset/1 -> Add3/2
  Brk_Liquid_Prs_mv/1 -> Divide3/1
  Add1/1 -> Saturation1/1
  Divide1/1 -> Add1/1
  Brk_Liquid_Prs_Factor/1 -> Divide3/2
  Divide/1 -> Add/1
  Add/1 -> Saturation/1
  Constant/1 -> Divide/2
  Acc_Right_Disp_mv/1 -> Divide1/1
  Acc_Lft_Disp_mv/1 -> Divide/1
  Gain/1 -> Saturation2/1
  Saturation2/1 -> Acc_Right_Disp_Val/1

== system FSAC2021_V1_Running/Input_Process/KL_Sig_Process/Whl_Spd_Process ==
  FL_WhlSpd_Hz : Inport
  FR_WhlSpd_Hz : Inport  Port=2
  RL_WhlSpd_Hz : Inport  Port=3
  RR_WhlSpd_Hz : Inport  Port=4
  LPF : Subsystem  TreatAsAtomicUnit=on
  LPF1 : Subsystem  TreatAsAtomicUnit=on
  LPF2 : Subsystem  TreatAsAtomicUnit=on
  LPF3 : Subsystem  TreatAsAtomicUnit=on
  MeaModule : ec55xxlib/RapidECU_U2/11Calibration/MeaModule  signal=Vel_spd
  Whl2Veh_Spd_Trans : Subsystem
  Whl_Spd_Hz2RPM : Subsystem  TreatAsAtomicUnit=on
  Whl_Spd_Hz2RPM1 : Subsystem  TreatAsAtomicUnit=on
  Whl_Spd_Hz2RPM2 : Subsystem  TreatAsAtomicUnit=on
  Whl_Spd_Hz2RPM3 : Subsystem  TreatAsAtomicUnit=on
  Vel_Spd : Outport
  Whl_Spd_FL_Val : Outport  Port=2
  Whl_Spd_FF_Val : Outport  Port=3
  Whl_Spd_RL_Val : Outport  Port=4
  Whl_Spd_RR_Val : Outport  Port=5
  wires:
  LPF3/1(Filtered) -> Whl2Veh_Spd_Trans/4(Wheel_speed_leftfront_wheel), Whl_Spd_RR_Val/1
  RR_WhlSpd_Hz/1 -> Whl_Spd_Hz2RPM3/1(Whl_Spd_Hz)
  RL_WhlSpd_Hz/1 -> Whl_Spd_Hz2RPM2/1(Whl_Spd_Hz)
  FR_WhlSpd_Hz/1 -> Whl_Spd_Hz2RPM1/1(Whl_Spd_Hz)
  FL_WhlSpd_Hz/1 -> Whl_Spd_Hz2RPM/1(Whl_Spd_Hz)
  Whl_Spd_Hz2RPM/1(Whl_Spd_RPM) -> LPF/1(Filter)
  LPF2/1(Filtered) -> Whl2Veh_Spd_Trans/3(Wheel_speed_leftrear_wheel), Whl_Spd_RL_Val/1
  LPF1/1(Filtered) -> Whl2Veh_Spd_Trans/2(Wheel_speed_right_front_wheel), Whl_Spd_FF_Val/1
  LPF/1(Filtered) -> Whl2Veh_Spd_Trans/1(Wheel_speed_rightrear_wheel), Whl_Spd_FL_Val/1
  Whl_Spd_Hz2RPM2/1(Whl_Spd_RPM) -> LPF2/1(Filter)
  Whl_Spd_Hz2RPM3/1(Whl_Spd_RPM) -> LPF3/1(Filter)
  Whl2Veh_Spd_Trans/1(Vel_Speed) -> MeaModule/1
  Whl_Spd_Hz2RPM1/1(Whl_Spd_RPM) -> LPF1/1(Filter)
  MeaModule/1 -> Vel_Spd/1

== system FSAC2021_V1_Running/ROUTING/TO_ACAN/DV_driving_dynamics_1 ==
  Streeing_angle_target_in : Inport
  Streeing_angle_actual_in : Inport  Port=2
  Speeed_target_in : Inport  Port=3
  Motor_moment_target_in : Inport  Port=4
  Motor_moment_actual_in : Inport  Port=5
  Brake_hydr_target_in : Inport  Port=6
  Brake_hydr_actual_in : Inport  Port=7
  Speeed_actual_in : Inport  Port=8
  Brake_hydr_actual : Subsystem
  Brake_hydr_target : Subsystem
  Conv{1..8} (8 alike) : DataTypeConversion
  DV_driving_dynamics_1_mux : Mux  Inputs=8
  Motor_moment_actual : Subsystem
  Motor_moment_target : Subsystem
  Speeed_actual : Subsystem
  Speeed_target : Subsystem
  Streeing_angle_actual : Subsystem
  Streeing_angle_target : Subsystem
  output : Outport
  wires:
  DV_driving_dynamics_1_mux/1 -> output/1
  Motor_moment_target/1(output8) -> Conv8/1
  Speeed_actual/1(output1) -> Conv1/1
  Conv1/1 -> DV_driving_dynamics_1_mux/1
  Speeed_target/1(output2) -> Conv2/1
  Conv2/1 -> DV_driving_dynamics_1_mux/2
  Streeing_angle_actual/1(output3) -> Conv3/1
  Conv3/1 -> DV_driving_dynamics_1_mux/3
  Streeing_angle_target/1(output4) -> Conv4/1
  Conv4/1 -> DV_driving_dynamics_1_mux/4
  Brake_hydr_actual/1(output5) -> Conv5/1
  Conv5/1 -> DV_driving_dynamics_1_mux/5
  Brake_hydr_target/1(output6) -> Conv6/1
  Conv6/1 -> DV_driving_dynamics_1_mux/6
  Motor_moment_actual/1(output7) -> Conv7/1
  Conv7/1 -> DV_driving_dynamics_1_mux/7
  Conv8/1 -> DV_driving_dynamics_1_mux/8
  Streeing_angle_target_in/1 -> Streeing_angle_target/1(Streeing_angle_target)
  Streeing_angle_actual_in/1 -> Streeing_angle_actual/1(Streeing_angle_actual)
  Speeed_target_in/1 -> Speeed_target/1(Speeed_target)
  Motor_moment_target_in/1 -> Motor_moment_target/1(Motor_moment_target)
  Motor_moment_actual_in/1 -> Motor_moment_actual/1(Motor_moment_actual)
  Brake_hydr_target_in/1 -> Brake_hydr_target/1(Brake_hydr_target)
  Brake_hydr_actual_in/1 -> Brake_hydr_actual/1(Brake_hydr_actual)
  Speeed_actual_in/1 -> Speeed_actual/1(Speeed_actual)

== system FSAC2021_V1_Running/ROUTING/TO_ACAN/DV_driving_dynamics_2 ==
  Yaw_rate_in : Inport
  Acceleration_longitudinal_in : Inport  Port=2
  Acceleration_lateral_in : Inport  Port=3
  Acceleration_lateral : Subsystem
  Acceleration_longitudinal : Subsystem
  Conv{1..6} (6 alike) : DataTypeConversion
  DV_driving_dynamics_2_mux : Mux  Inputs=6
  Yaw_rate : Subsystem
  output : Outport
  wires:
  DV_driving_dynamics_2_mux/1 -> output/1
  Acceleration_longitudinal/1(output1) -> Conv1/1
  Conv1/1 -> DV_driving_dynamics_2_mux/1
  Acceleration_longitudinal/2(output2) -> Conv2/1
  Conv2/1 -> DV_driving_dynamics_2_mux/2
  Yaw_rate/1(output3) -> Conv3/1
  Conv3/1 -> DV_driving_dynamics_2_mux/3
  Yaw_rate/2(output4) -> Conv4/1
  Conv4/1 -> DV_driving_dynamics_2_mux/4
  Acceleration_lateral/1(output5) -> Conv5/1
  Conv5/1 -> DV_driving_dynamics_2_mux/5
  Acceleration_lateral/2(output6) -> Conv6/1
  Conv6/1 -> DV_driving_dynamics_2_mux/6
  Yaw_rate_in/1 -> Yaw_rate/1(Yaw_rate)
  Acceleration_longitudinal_in/1 -> Acceleration_longitudinal/1(Acceleration_longitudinal)
  Acceleration_lateral_in/1 -> Acceleration_lateral/1(Acceleration_lateral)

== system FSAC2021_V1_Running/ROUTING/TO_ACAN/DV_system_status ==
  Steering_state_in : Inport
  Service_brake_state_in : Inport  Port=2
  Lap_counter_in : Inport  Port=3
  EBS_State_in : Inport  Port=4
  Cones_count_all_in : Inport  Port=5
  Cones_count_actual_in : Inport  Port=6
  ASSI_State_in : Inport  Port=7
  AMI_State_in : Inport  Port=8
  AMI_State : Subsystem
  ASSI_State : Subsystem
  Cones_count_actual : Subsystem
  Cones_count_all : Subsystem
  Conv{1..5} (5 alike) : DataTypeConversion
  DV_system_status_mux : Mux  Inputs=5
  EBS_State : Subsystem
  Lap_counter : Subsystem
  Service_brake_state : Subsystem
  Steering_state : Subsystem
  or1 : simulink/Logic and Bit Operations/Bitwise Operator  logicop=OR  UseBitMask=off  NumInputPorts=3  BitMask=bin2dec('11011001')  BitMaskRealWorld=Stored Integer
  or2 : simulink/Logic and Bit Operations/Bitwise Operator  logicop=OR  UseBitMask=off  NumInputPorts=4  BitMask=bin2dec('11011001')  BitMaskRealWorld=Stored Integer
  or3 : simulink/Logic and Bit Operations/Bitwise Operator  logicop=OR  UseBitMask=off  NumInputPorts=2  BitMask=bin2dec('11011001')  BitMaskRealWorld=Stored Integer
  output : Outport
  wires:
  DV_system_status_mux/1 -> output/1
  Steering_state/1(output2) -> or2/1
  Service_brake_state/1(output2) -> or2/2
  Lap_counter/1(output2) -> or2/3
  EBS_State/1(output1) -> or1/1
  Cones_count_all/1(output3) -> or3/2
  Cones_count_actual/1(output2) -> or2/4
  Cones_count_actual/2(output3) -> or3/1
  ASSI_State/1(output1) -> or1/2
  AMI_State/1(output1) -> or1/3
  or1/1 -> Conv1/1
  Conv1/1 -> DV_system_status_mux/1
  or2/1 -> Conv2/1
  Conv2/1 -> DV_system_status_mux/2
  or3/1 -> Conv3/1
  Conv3/1 -> DV_system_status_mux/3
  Cones_count_all/2(output4) -> Conv4/1
  Conv4/1 -> DV_system_status_mux/4
  Cones_count_all/3(output5) -> Conv5/1
  Conv5/1 -> DV_system_status_mux/5
  Steering_state_in/1 -> Steering_state/1(Steering_state)
  Service_brake_state_in/1 -> Service_brake_state/1(Service_brake_state)
  Lap_counter_in/1 -> Lap_counter/1(Lap_counter)
  EBS_State_in/1 -> EBS_State/1(EBS_State)
  Cones_count_all_in/1 -> Cones_count_all/1(Cones_count_all)
  Cones_count_actual_in/1 -> Cones_count_actual/1(Cones_count_actual)
  ASSI_State_in/1 -> ASSI_State/1(ASSI_State)
  AMI_State_in/1 -> AMI_State/1(AMI_State)
